simulink model "SRM"  (R2013b)
settings: Solver=ode8  StartTime=0.0  StopTime=2  FixedStep=Ts  RelTol=1e-3
InitFcn:
  | Iref=4
  | v_4dc = 78;
  | kp_speed =500;
  | ki_speed = 60;
  | sat_speed = 10;
  | x = 0.8 ;%%firing angle
  | kp_controller = 200;
  | ki_controller = 60;
  | ts = 1/10e4;
  | Ts = 1e-06;
undefined symbols (not defined in the file): find_system
libraries: simulink x1, powerlib x1
settings Model: Creator=Mircea Ruba  LastModifiedBy=agie
settings DataIOCC: SignalLoggingSaveFormat=ModelDataLogs
settings OptimizationCC: ExpressionDepthLimit=2147483647
settings DebuggingCC: FcnCallInpInsideContextMsg=UseLocalSettings  UnconnectedInputMsg=none  UnconnectedOutputMsg=none  UnconnectedLineMsg=none  StateNameClashWarn=warning
settings GRTTargetCC: CombineOutputUpdateFcns=off  GRTInterface=on
settings ConfigurationSet: Description=SimMechanics 2G

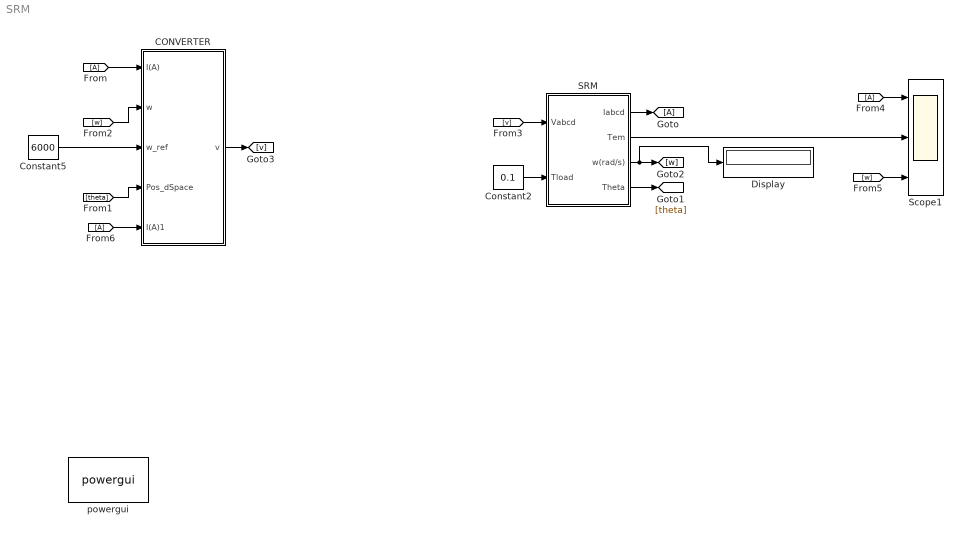
== system SRM ==
  CONVERTER : Subsystem  LoadFcn=find_system(gcs,'FollowLinks', 'on', 'LookUnderMasks', 'all');
  Constant2 : Constant  Value=0.1
  Constant5 : Constant  Value=6000
  Display : Display
  SRM : Subsystem
  Scope1 : Scope  NumInputPorts=3
      settings: TimeRange=0.5  YMin=-1~5.55112e-17~0  YMax=12~1~1100
  powergui : powerlib/powergui  Priority=2  SimulationMode=Discrete  SolverType=Tustin  SampleTime=Ts  frequency=60  SPID=off  DisableSnubberDevices=off  DisableRonSwitches=off  DisableVfSwitches=off  SwTol=0  Interpol=off  DisplayEquations=off  frequencyindice=0  Pbase=100e6  ErrMax=1e-4  Iterations=50  UnitsV=kV  UnitsW=MW  FunctionMessages=off  echomessages=off  HookPort=off  EnableUseOfTLC=off  x0status=blocks  RestoreLinks=warning  ResistiveCurrentMeasurement=off  Frange=[0:2:500]  Ylog=off  Xlog=on  ShowGrid=off  save=off  variable=ZData  ZoomFFT=on  StartTime=0.0  cycles=1  DisplayStyle=1  fundamental=60  FreqAxis=off  MaxFrequency=1000  frequencyindicesteady=1  RmsSteady=1  display=off  Ts=0  methode=off
  wires:
  SRM/2(Tem) -> Scope1/2
  Constant2/1 -> SRM/2(Tload)
  Constant5/1 -> CONVERTER/3(w_ref)
  SRM/1(Iabcd) -> [A]
  [A] -> CONVERTER/1(I(A))
  SRM/4(Theta) -> [theta]
  [theta] -> CONVERTER/4(Pos_dSpace)
  SRM/3(w(rad/s)) -> Display/1, [w]
  [w] -> CONVERTER/2(w)
  CONVERTER/1(v) -> [v]
  [v] -> SRM/1(Vabcd)
  [A] -> Scope1/1
  [w] -> Scope1/3
  [A] -> CONVERTER/5(I(A)1)

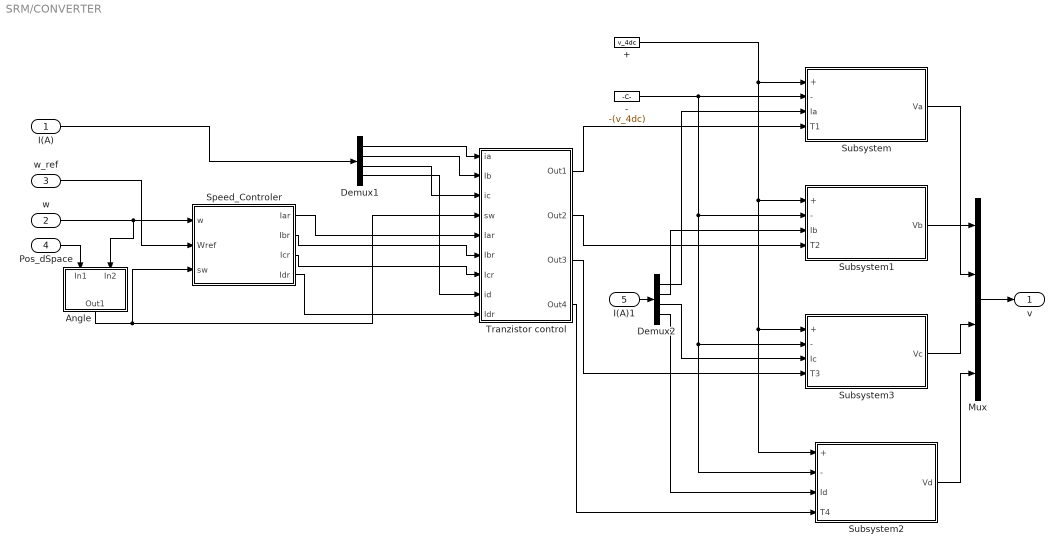
== system SRM/CONVERTER ==
  I(A) : Inport
  w : Inport  Port=2
  w_ref : Inport  Port=3
  Pos_dSpace : Inport  Port=4
  I(A)1 : Inport  Port=5
  + : Constant  Value=v_4dc
  - : Constant  Value=-(v_4dc)
  Angle : Subsystem
  Demux1 : Demux
  Demux2 : Demux
  Mux : Mux
  Speed_Controler : Subsystem
  Subsystem : Subsystem
  Subsystem1 : Subsystem
  Subsystem2 : Subsystem
  Subsystem3 : Subsystem
  Tranzistor control : Subsystem
  v : Outport
  wires:
  Demux1/4 -> Tranzistor control/8(id)
  Speed_Controler/4(Idr) -> Tranzistor control/9(Idr)
  Speed_Controler/1(Iar) -> Tranzistor control/5(Iar)
  Speed_Controler/2(Ibr) -> Tranzistor control/6(Ibr)
  Speed_Controler/3(Icr) -> Tranzistor control/7(Icr)
  Demux1/1 -> Tranzistor control/1(ia)
  Demux1/2 -> Tranzistor control/2(Ib)
  Demux1/3 -> Tranzistor control/3(ic)
  I(A)/1 -> Demux1/1
  w_ref/1 -> Speed_Controler/2(Wref)
  w/1 -> Speed_Controler/1(w), Angle/2(In2)
  Mux/1 -> v/1
  +/1 -> Subsystem2/1(+), Subsystem3/1(+), Subsystem1/1(+), Subsystem/1(+)
  -/1 -> Subsystem2/2(-), Subsystem3/2(-), Subsystem1/2(-), Subsystem/2(-)
  Angle/1(Out1) -> Speed_Controler/3("sw "), Tranzistor control/4("sw ")
  Pos_dSpace/1 -> Angle/1(In1)
  Tranzistor control/1(Out1) -> Subsystem/4(T1)
  Subsystem/1(Va) -> Mux/1
  Tranzistor control/2(Out2) -> Subsystem1/4(T2)
  Subsystem1/1(Vb) -> Mux/2
  Tranzistor control/4(Out4) -> Subsystem2/4(T4)
  Subsystem2/1(Vd) -> Mux/4
  Tranzistor control/3(Out3) -> Subsystem3/4(T3)
  Subsystem3/1(Vc) -> Mux/3
  I(A)1/1 -> Demux2/1
  Demux2/1 -> Subsystem/3(Ia)
  Demux2/2 -> Subsystem1/3(Ib)
  Demux2/3 -> Subsystem3/3(Ic)
  Demux2/4 -> Subsystem2/3(Id)

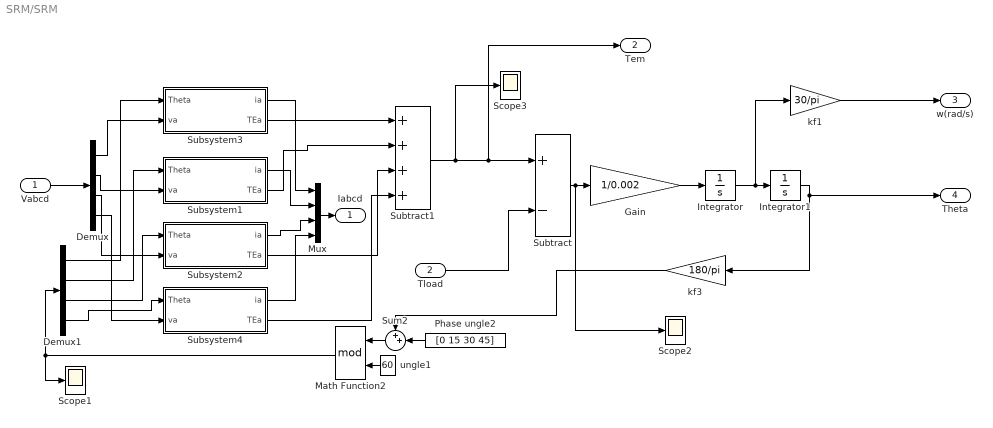
== system SRM/SRM ==
  Vabcd : Inport
  Tload : Inport  Port=2
  Demux : Demux
  Demux1 : Demux
  Gain : Gain  Gain=1/0.002
  Integrator : Integrator
  Integrator1 : Integrator  InitialCondition=10
  Math Function2 : Math  Operator=mod  SaturateOnIntegerOverflow=on
  Mux : Mux
  Phase ungle2 : Constant  Value=[0 15 30 45]
  Scope1 : Scope
      settings: TimeRange=0.4368  YMin=0  YMax=60
  Scope2 : Scope
      settings: TimeRange=0.4368  YMin=-550  YMax=300  SaveName=ScopeData11
  Scope3 : Scope
      settings: TimeRange=0.4368  YMin=-450  YMax=400  SaveName=ScopeData9
  Subsystem1 : Subsystem
  Subsystem2 : Subsystem
  Subsystem3 : Subsystem
  Subsystem4 : Subsystem
  Subtract : Sum  Inputs=+-
  Subtract1 : Sum  Inputs=++++
  Sum2 : Sum  Inputs=++|  SaturateOnIntegerOverflow=on  InputSameDT=on  OutDataTypeStr=Inherit: Same as first input
  kf1 : Gain  Gain=30/pi
  kf3 : Gain  Gain=180/pi
  ungle1 : Constant  Value=60
  Iabcd : Outport
  Tem : Outport  Port=2
  w(rad/s) : Outport  Port=3
  Theta : Outport  Port=4
  wires:
  Demux/4 -> Subsystem4/2(va)
  Demux1/4 -> Subsystem4/1(Theta)
  Subsystem4/2(TEa) -> Subtract1/4
  Subsystem4/1(ia) -> Mux/4
  Math Function2/1 -> Scope1/1, Demux1/1
  ungle1/1 -> Math Function2/2
  Sum2/1 -> Math Function2/1
  Phase ungle2/1 -> Sum2/2
  Vabcd/1 -> Demux/1
  Demux/1 -> Subsystem3/2(va)
  Mux/1 -> Iabcd/1
  Subsystem3/1(ia) -> Mux/1
  Subsystem1/1(ia) -> Mux/2
  Subsystem2/1(ia) -> Mux/3
  Subsystem2/2(TEa) -> Subtract1/3
  Subsystem1/2(TEa) -> Subtract1/2
  Subsystem3/2(TEa) -> Subtract1/1
  Subtract1/1 -> Subtract/1, Tem/1, Scope3/1
  Gain/1 -> Integrator/1
  Subtract/1 -> Scope2/1, Gain/1
  Integrator1/1 -> Theta/1, kf3/1
  Demux/2 -> Subsystem1/2(va)
  Demux/3 -> Subsystem2/2(va)
  Tload/1 -> Subtract/2
  kf3/1 -> Sum2/1
  Demux1/1 -> Subsystem3/1(Theta)
  Demux1/2 -> Subsystem1/1(Theta)
  Demux1/3 -> Subsystem2/1(Theta)
  Integrator/1 -> kf1/1, Integrator1/1
  kf1/1 -> w(rad/s)/1

== system SRM/CONVERTER/Angle ==
  In1 : Inport
  In2 : Inport  Port=2
  360 : Subsystem
  Position : Subsystem
  angle : Subsystem
  Out1 : Outport
  wires:
  Position/1(sw) -> Out1/1
  angle/1(Theta_On(Alpha)) -> Position/2(On angle)
  angle/2(Theta_Off(Beta)) -> Position/3(Off angle)
  In1/1 -> 360/1(In1)
  In2/1 -> angle/1(n)
  360/1(Out1) -> Position/1(dSpace POSITION)

== system SRM/CONVERTER/Speed_Controler ==
  w : Inport
  Wref : Inport  Port=2
  "sw " : Inport  Port=3
  Add : Sum  Inputs=+-
  Demux : Demux
  PI+AntiWindup : Subsystem
  Product{,1..3} (4 alike) : Product
  Iar : Outport
  Ibr : Outport  Port=2
  Icr : Outport  Port=3
  Idr : Outport  Port=4
  wires:
  Product3/1 -> Idr/1
  PI+AntiWindup/1(Out) -> Product2/1, Product3/1, Product1/1, Product/1
  Demux/4 -> Product3/2
  w/1 -> Add/2
  Wref/1 -> Add/1
  Product/1 -> Iar/1
  "sw "/1 -> Demux/1
  Product1/1 -> Ibr/1
  Product2/1 -> Icr/1
  Add/1 -> PI+AntiWindup/1(In)
  Demux/1 -> Product/2
  Demux/2 -> Product1/2
  Demux/3 -> Product2/2

== system SRM/CONVERTER/Subsystem ==
  + : Inport
  - : Inport  Port=2
  Ia : Inport  Port=3
  T1 : Inport  Port=4
  Constant5 : Constant  Value=0
  Switch : Switch  Criteria=u2 > Threshold  SaturateOnIntegerOverflow=on  InputSameDT=on
  Switch5 : Switch  Criteria=u2 > Threshold  SaturateOnIntegerOverflow=on  InputSameDT=on
  Va : Outport
  wires:
  +/1 -> Switch/1
  Ia/1 -> Switch5/2
  -/1 -> Switch5/1
  T1/1 -> Switch/2
  Constant5/1 -> Switch5/3
  Switch5/1 -> Switch/3
  Switch/1 -> Va/1

== system SRM/CONVERTER/Subsystem1 ==
  + : Inport
  - : Inport  Port=2
  Ib : Inport  Port=3
  T2 : Inport  Port=4
  Constant2 : Constant  Value=0
  Switch1 : Switch  Criteria=u2 > Threshold  SaturateOnIntegerOverflow=on  InputSameDT=on
  Switch2 : Switch  Criteria=u2 > Threshold  SaturateOnIntegerOverflow=on  InputSameDT=on
  Vb : Outport
  wires:
  Switch2/1 -> Switch1/3
  Constant2/1 -> Switch2/3
  T2/1 -> Switch1/2
  Switch1/1 -> Vb/1
  Ib/1 -> Switch2/2
  -/1 -> Switch2/1
  +/1 -> Switch1/1

== system SRM/CONVERTER/Subsystem2 ==
  + : Inport
  - : Inport  Port=2
  Id : Inport  Port=3
  T4 : Inport  Port=4
  Constant4 : Constant  Value=0
  Switch6 : Switch  Criteria=u2 > Threshold  SaturateOnIntegerOverflow=on  InputSameDT=on
  Switch7 : Switch  Criteria=u2 > Threshold  SaturateOnIntegerOverflow=on  InputSameDT=on
  Vd : Outport
  wires:
  T4/1 -> Switch6/2
  Switch6/1 -> Vd/1
  Constant4/1 -> Switch7/3
  Switch7/1 -> Switch6/3
  +/1 -> Switch6/1
  Id/1 -> Switch7/2
  -/1 -> Switch7/1

== system SRM/CONVERTER/Subsystem3 ==
  + : Inport
  - : Inport  Port=2
  Ic : Inport  Port=3
  T3 : Inport  Port=4
  Constant3 : Constant  Value=0
  Switch3 : Switch  Criteria=u2 > Threshold  SaturateOnIntegerOverflow=on  InputSameDT=on
  Switch4 : Switch  Criteria=u2 > Threshold  SaturateOnIntegerOverflow=on  InputSameDT=on
  Vc : Outport
  wires:
  Ic/1 -> Switch4/2
  +/1 -> Switch3/1
  -/1 -> Switch4/1
  T3/1 -> Switch3/2
  Switch3/1 -> Vc/1
  Constant3/1 -> Switch4/3
  Switch4/1 -> Switch3/3

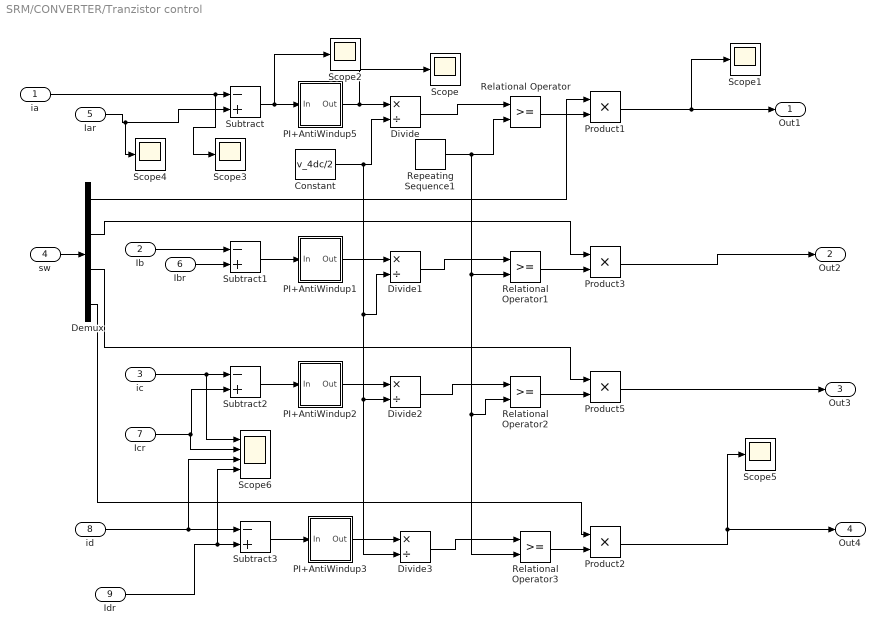
== system SRM/CONVERTER/Tranzistor control ==
  ia : Inport
  Ib : Inport  Port=2
  ic : Inport  Port=3
  "sw " : Inport  Port=4
  Iar : Inport  Port=5
  Ibr : Inport  Port=6
  Icr : Inport  Port=7
  id : Inport  Port=8
  Idr : Inport  Port=9
  Constant : Constant  Value=v_4dc/2
  Demux : Demux
  Divide{,1..3} (4 alike) : Product  Inputs=*/
  PI+AntiWindup1 : Subsystem
  PI+AntiWindup2 : Subsystem
  PI+AntiWindup3 : Subsystem
  PI+AntiWindup5 : Subsystem
  Product{1..3,5} (4 alike) : Product
  Relational Operator{,1..3} (4 alike) : RelationalOperator  OutDataTypeStr=boolean
  Repeating Sequence1 : simulink/Sources/Repeating Sequence  rep_seq_t=[0 0.5 1]*(1/10e3)  rep_seq_y=[-0.999 0.999 -0.999]
  Scope{,1..5} (6 alike) : Scope
      Scope settings: YMin=-45  YMax=45  SaveName=ScopeData10
      Scope1 settings: YMin=-45  YMax=45  SaveName=ScopeData16
      Scope2 settings: YMin=-5.5  YMax=5.5  SaveName=ScopeData17
      Scope3 settings: YMin=-0.008  YMax=-0.001  SaveName=ScopeData19
      Scope4 settings: YMin=-5.5  YMax=5.5  SaveName=ScopeData21
      Scope5 settings: YMin=-45  YMax=45  SaveName=ScopeData22
  Scope6 : Scope  NumInputPorts=4
      settings: YMin=-250~0~-80~0  YMax=50~5~10~5  SaveName=ScopeData23
  Subtract{,1..3} (4 alike) : Sum  Inputs=-+
  Out1 : Outport
  Out2 : Outport  Port=2
  Out3 : Outport  Port=3
  Out4 : Outport  Port=4
  wires:
  Product2/1 -> Scope5/1, Out4/1
  Constant/1 -> Divide/2, Divide3/2, Divide2/2, Divide1/2
  Divide3/1 -> Relational Operator3/1
  PI+AntiWindup3/1(Out) -> Divide3/1
  id/1 -> Scope6/3, Subtract3/1
  Idr/1 -> Scope6/4, Subtract3/2
  Subtract3/1 -> PI+AntiWindup3/1(In)
  Relational Operator3/1 -> Product2/2
  Demux/4 -> Product2/1
  Repeating Sequence1/1 -> Relational Operator/2, Relational Operator1/2, Relational Operator2/2, Relational Operator3/2
  Divide2/1 -> Relational Operator2/1
  PI+AntiWindup2/1(Out) -> Divide2/1
  Divide1/1 -> Relational Operator1/1
  PI+AntiWindup1/1(Out) -> Divide1/1
  PI+AntiWindup5/1(Out) -> Divide/1, Scope/1
  Divide/1 -> Relational Operator/1
  Iar/1 -> Scope4/1, Subtract/2
  Relational Operator/1 -> Product1/2
  Ib/1 -> Subtract1/1
  Ibr/1 -> Subtract1/2
  Subtract1/1 -> PI+AntiWindup1/1(In)
  Relational Operator1/1 -> Product3/2
  Product3/1 -> Out2/1
  ic/1 -> Scope6/1, Subtract2/1
  Icr/1 -> Scope6/2, Subtract2/2
  Subtract2/1 -> PI+AntiWindup2/1(In)
  Relational Operator2/1 -> Product5/2
  Product5/1 -> Out3/1
  Demux/1 -> Product1/1
  Demux/2 -> Product3/1
  Demux/3 -> Product5/1
  "sw "/1 -> Demux/1
  Product1/1 -> Scope1/1, Out1/1
  Subtract/1 -> Scope2/1, PI+AntiWindup5/1(In)
  ia/1 -> Scope3/1, Subtract/1

== system SRM/SRM/Subsystem1 ==
  Theta : Inport
  va : Inport  Port=2
  Gain : Gain  Gain=0.3
  Product : Product
  Product1 : Product
  Scope4 : Scope  NumInputPorts=3
      settings: TimeRange=0.5  YMin=-1~-1~-25  YMax=1~1~25  SaveName=ScopeData20
  "Subsystem2 " : Subsystem
  Sum : Sum  Inputs=|+-
  ia : Outport
  TEa : Outport  Port=2
  wires:
  va/1 -> Sum/1
  Sum/1 -> "Subsystem2 "/2(Lambda)
  "Subsystem2 "/2(Current) -> ia/1, Gain/1, Product1/2, Product1/1
  Gain/1 -> Sum/2
  Product1/1 -> Product/2, Scope4/2
  "Subsystem2 "/1(dL/dt) -> Product/1, Scope4/1
  Product/1 -> Scope4/3, TEa/1
  Theta/1 -> "Subsystem2 "/1(Theta)

== system SRM/SRM/Subsystem2 ==
  Theta : Inport
  va : Inport  Port=2
  Gain : Gain  Gain=0.3
  Product : Product
  Product1 : Product
  Scope4 : Scope  NumInputPorts=3
      settings: TimeRange=0.5  YMin=-1~-1~-25  YMax=1~1~25  SaveName=ScopeData20
  "Subsystem2 " : Subsystem
  Sum : Sum  Inputs=|+-
  ia : Outport
  TEa : Outport  Port=2
  wires:
  Theta/1 -> "Subsystem2 "/1(Theta)
  Product/1 -> TEa/1, Scope4/3
  "Subsystem2 "/1(dL/dt) -> Scope4/1, Product/1
  Product1/1 -> Product/2, Scope4/2
  Gain/1 -> Sum/2
  "Subsystem2 "/2(Current) -> Product1/1, Product1/2, Gain/1, ia/1
  Sum/1 -> "Subsystem2 "/2(Lambda)
  va/1 -> Sum/1

== system SRM/SRM/Subsystem3 ==
  Theta : Inport
  va : Inport  Port=2
  Gain : Gain  Gain=0.3
  Product : Product
  Product1 : Product
  "Subsystem2 " : Subsystem
  Sum : Sum  Inputs=|+-
  ia : Outport
  TEa : Outport  Port=2
  wires:
  Theta/1 -> "Subsystem2 "/1(Theta)
  Product/1 -> TEa/1
  "Subsystem2 "/1(dL/dt) -> Product/1
  Product1/1 -> Product/2
  Gain/1 -> Sum/2
  "Subsystem2 "/2(Current) -> Product1/1, Product1/2, Gain/1, ia/1
  Sum/1 -> "Subsystem2 "/2(Lambda)
  va/1 -> Sum/1

== system SRM/SRM/Subsystem4 ==
  Theta : Inport
  va : Inport  Port=2
  Gain : Gain
  Product : Product
  Product1 : Product
  Scope4 : Scope  NumInputPorts=3
      settings: TimeRange=0.5  YMin=-1~-1~-25  YMax=1~1~25  SaveName=ScopeData20
  "Subsystem2 " : Subsystem
  Sum : Sum  Inputs=|+-
  ia : Outport
  TEa : Outport  Port=2
  wires:
  va/1 -> Sum/1
  Sum/1 -> "Subsystem2 "/2(Lambda)
  "Subsystem2 "/2(Current) -> Scope4/2, ia/1, Gain/1, Product1/2, Product1/1
  Gain/1 -> Sum/2
  Product1/1 -> Product/2
  "Subsystem2 "/1(dL/dt) -> Scope4/1, Product/1
  Product/1 -> Scope4/3, TEa/1
  Theta/1 -> "Subsystem2 "/1(Theta)

== system SRM/CONVERTER/Angle/360 ==
  In1 : Inport
  Constant2 : Constant  Value=360
  Math Function2 : Math  Operator=mod  SaturateOnIntegerOverflow=on
  kf2 : Gain  Gain=180/pi
  Out1 : Outport
  wires:
  Constant2/1 -> Math Function2/2
  kf2/1 -> Math Function2/1
  Math Function2/1 -> Out1/1
  In1/1 -> kf2/1

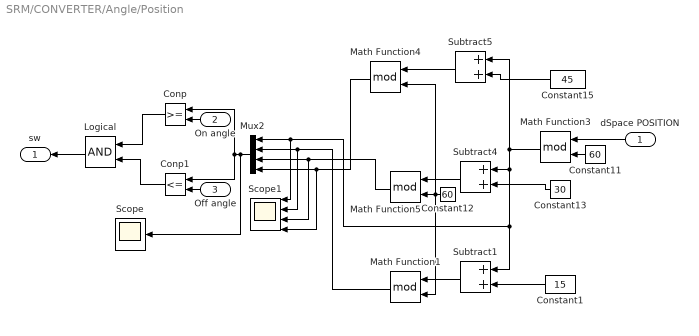
== system SRM/CONVERTER/Angle/Position ==
  dSpace POSITION : Inport
  On angle : Inport  Port=2
  Off angle : Inport  Port=3
  " Logical" : Logic  AllPortsSameDT=off  OutDataTypeStr=boolean
  Conp : RelationalOperator  OutDataTypeStr=boolean
  Conp1 : RelationalOperator  Operator=<=  OutDataTypeStr=boolean
  Constant1 : Constant  Value=15
  Constant11 : Constant  Value=60
  Constant12 : Constant  Value=60
  Constant13 : Constant  Value=30
  Constant15 : Constant  Value=45
  Math Function{1,3..5} (4 alike) : Math  Operator=mod  SaturateOnIntegerOverflow=on
  Mux2 : Mux
  Scope : Scope
      settings: YMin=10  YMax=75  SaveName=ScopeData14
  Scope1 : Scope  NumInputPorts=4
      settings: YMin=10~-5~-5~-5  YMax=75~5~5~5  SaveName=ScopeData3
  Subtract1 : Sum
  Subtract4 : Sum
  Subtract5 : Sum
  sw : Outport
  wires:
  Math Function1/1 -> Scope1/2, Mux2/2
  Constant1/1 -> Subtract1/2
  Subtract1/1 -> Math Function1/1
  Constant11/1 -> Math Function3/2
  Math Function3/1 -> Subtract1/1, Mux2/1, Scope1/1, Subtract4/1, Subtract5/1
  Subtract4/1 -> Math Function5/1
  Constant13/1 -> Subtract4/2
  Subtract5/1 -> Math Function4/1
  dSpace POSITION/1 -> Math Function3/1
  Constant15/1 -> Subtract5/2
  Math Function4/1 -> Mux2/4, Scope1/4
  Constant12/1 -> Math Function4/2, Math Function5/2, Math Function1/2
  Math Function5/1 -> Mux2/3, Scope1/3
  Mux2/1 -> Scope/1, Conp/1, Conp1/1
  Conp/1 -> " Logical"/1
  Conp1/1 -> " Logical"/2
  " Logical"/1 -> sw/1
  On angle/1 -> Conp/2
  Off angle/1 -> Conp1/2

== system SRM/CONVERTER/Angle/angle ==
  n : Inport
  Iref1 : Constant  Value=Iref
  Subsystem : Subsystem
  Subsystem1 : Subsystem
  Theta_On(Alpha) : Outport
  Theta_Off(Beta) : Outport  Port=2
  wires:
  Subsystem/1(Theta_ON) -> Theta_On(Alpha)/1
  Subsystem1/1(Theta_Off) -> Theta_Off(Beta)/1
  Iref1/1 -> Subsystem1/1(Iref), Subsystem/1(Iref)
  n/1 -> Subsystem1/2(n), Subsystem/2(n)

== system SRM/CONVERTER/Speed_Controler/PI+AntiWindup ==
  In : Inport
  Gain10 : Gain  Gain=ki_speed
  Gain11 : Gain  Gain=1/kp_speed
  Gain9 : Gain  Gain=kp_speed
  Integrator3 : Integrator
  Saturation3 : Saturate  UpperLimit=sat_speed  LowerLimit=-sat_speed
  Sum10 : Sum  Inputs=|++
  Sum11 : Sum  Inputs=-+|
  Sum9 : Sum
  Out : Outport
  wires:
  Sum9/1 -> Integrator3/1
  Integrator3/1 -> Gain10/1
  Gain9/1 -> Sum10/1
  Sum11/1 -> Gain11/1
  In/1 -> Sum9/1, Gain9/1
  Saturation3/1 -> Out/1, Sum11/2
  Sum10/1 -> Saturation3/1, Sum11/1
  Gain11/1 -> Sum9/2
  Gain10/1 -> Sum10/2

== system SRM/CONVERTER/Tranzistor control/PI+AntiWindup1 ==
  In : Inport
  Gain10 : Gain  Gain=ki_controller
  Gain11 : Gain  Gain=1/kp_controller
  Gain9 : Gain  Gain=kp_controller
  Integrator3 : Integrator
  Saturation3 : Saturate  UpperLimit=v_4dc/2  LowerLimit=-v_4dc/2  LinearizeAsGain=off
  Sum10 : Sum  Inputs=|++
  Sum11 : Sum  Inputs=-+|
  Sum9 : Sum
  Out : Outport
  wires:
  Gain11/1 -> Sum9/2
  In/1 -> Gain9/1, Sum9/1
  Sum11/1 -> Gain11/1
  Sum10/1 -> Saturation3/1, Sum11/1
  Gain9/1 -> Sum10/1
  Gain10/1 -> Sum10/2
  Integrator3/1 -> Gain10/1
  Sum9/1 -> Integrator3/1
  Saturation3/1 -> Sum11/2, Out/1

== system SRM/CONVERTER/Tranzistor control/PI+AntiWindup2 ==
  In : Inport
  Gain10 : Gain  Gain=ki_controller
  Gain11 : Gain  Gain=1/kp_controller
  Gain9 : Gain  Gain=kp_controller
  Integrator3 : Integrator
  Saturation3 : Saturate  UpperLimit=v_4dc/2  LowerLimit=-v_4dc/2  LinearizeAsGain=off
  Sum10 : Sum  Inputs=|++
  Sum11 : Sum  Inputs=-+|
  Sum9 : Sum
  Out : Outport
  wires:
  Saturation3/1 -> Out/1, Sum11/2
  Sum9/1 -> Integrator3/1
  Integrator3/1 -> Gain10/1
  Gain10/1 -> Sum10/2
  Gain9/1 -> Sum10/1
  Sum10/1 -> Saturation3/1, Sum11/1
  Sum11/1 -> Gain11/1
  In/1 -> Sum9/1, Gain9/1
  Gain11/1 -> Sum9/2

== system SRM/CONVERTER/Tranzistor control/PI+AntiWindup3 ==
  In : Inport
  Gain10 : Gain  Gain=ki_controller
  Gain11 : Gain  Gain=1/kp_controller
  Gain9 : Gain  Gain=kp_controller
  Integrator3 : Integrator
  Saturation3 : Saturate  UpperLimit=v_4dc/2  LowerLimit=-v_4dc/2  LinearizeAsGain=off
  Sum10 : Sum  Inputs=|++
  Sum11 : Sum  Inputs=-+|
  Sum9 : Sum
  Out : Outport
  wires:
  Saturation3/1 -> Out/1, Sum11/2
  Sum9/1 -> Integrator3/1
  Integrator3/1 -> Gain10/1
  Gain10/1 -> Sum10/2
  Gain9/1 -> Sum10/1
  Sum10/1 -> Saturation3/1, Sum11/1
  Sum11/1 -> Gain11/1
  In/1 -> Sum9/1, Gain9/1
  Gain11/1 -> Sum9/2

== system SRM/CONVERTER/Tranzistor control/PI+AntiWindup5 ==
  In : Inport
  Gain10 : Gain  Gain=ki_controller
  Gain11 : Gain  Gain=1/kp_controller
  Gain9 : Gain  Gain=kp_controller
  Integrator3 : Integrator
  Saturation3 : Saturate  UpperLimit=v_4dc/2  LowerLimit=-v_4dc/2  LinearizeAsGain=off
  Scope : Scope  NumInputPorts=4
      settings: YMin=-5~-5000~0.2~-1500  YMax=5~45000~0.65~250  SaveName=ScopeData4
  Sum10 : Sum  Inputs=|++
  Sum11 : Sum  Inputs=-+|
  Sum9 : Sum
  Out : Outport
  wires:
  Saturation3/1 -> Scope/1, Out/1, Sum11/2
  Sum9/1 -> Integrator3/1
  Integrator3/1 -> Gain10/1
  Gain10/1 -> Sum10/2, Scope/4
  Gain9/1 -> Scope/3, Sum10/1
  Sum10/1 -> Scope/2, Saturation3/1, Sum11/1
  Sum11/1 -> Gain11/1
  In/1 -> Sum9/1, Gain9/1
  Gain11/1 -> Sum9/2

== system SRM/SRM/Subsystem1/Subsystem2  ==
  Theta : Inport
  Lambda : Inport  Port=2
  Divide : Product  Inputs=*/
  Integrator : Integrator
  Subsystem1 : Subsystem
  Subsystem2 : Subsystem
  dL/dt : Outport
  Current : Outport  Port=2
  wires:
  Subsystem1/1(dL/dt) -> dL/dt/1
  Theta/1 -> Subsystem2/1(Theta), Subsystem1/1(Theta)
  Lambda/1 -> Divide/1
  Subsystem2/1(L(theta)) -> Divide/2
  Divide/1 -> Integrator/1
  Integrator/1 -> Current/1

== system SRM/SRM/Subsystem2/Subsystem2  ==
  Theta : Inport
  Lambda : Inport  Port=2
  Divide : Product  Inputs=*/
  Integrator : Integrator
  Subsystem1 : Subsystem
  Subsystem2 : Subsystem
  dL/dt : Outport
  Current : Outport  Port=2
  wires:
  Divide/1 -> Integrator/1
  Subsystem2/1(L(theta)) -> Divide/2
  Lambda/1 -> Divide/1
  Theta/1 -> Subsystem1/1(Theta), Subsystem2/1(Theta)
  Subsystem1/1(dL/dt) -> dL/dt/1
  Integrator/1 -> Current/1

== system SRM/SRM/Subsystem3/Subsystem2  ==
  Theta : Inport
  Lambda : Inport  Port=2
  Divide : Product  Inputs=*/
  Integrator1 : Integrator
  Subsystem1 : Subsystem
  Subsystem2 : Subsystem
  dL/dt : Outport
  Current : Outport  Port=2
  wires:
  Divide/1 -> Integrator1/1
  Subsystem2/1(L(theta)) -> Divide/2
  Lambda/1 -> Divide/1
  Theta/1 -> Subsystem1/1(Theta), Subsystem2/1(Theta)
  Subsystem1/1(dL/dt) -> dL/dt/1
  Integrator1/1 -> Current/1

== system SRM/SRM/Subsystem4/Subsystem2  ==
  Theta : Inport
  Lambda : Inport  Port=2
  Divide : Product  Inputs=*/
  Integrator : Integrator
  Subsystem1 : Subsystem
  Subsystem2 : Subsystem
  dL/dt : Outport
  Current : Outport  Port=2
  wires:
  Subsystem1/1(dL/dt) -> dL/dt/1
  Theta/1 -> Subsystem2/1(Theta), Subsystem1/1(Theta)
  Lambda/1 -> Divide/1
  Subsystem2/1(L(theta)) -> Divide/2
  Divide/1 -> Integrator/1
  Integrator/1 -> Current/1

== system SRM/CONVERTER/Angle/angle/Subsystem ==
  Iref : Inport
  n : Inport  Port=2
  Dc link : Constant  Value=42
  Divide : Product  Inputs=*/
  Lu : Constant  Value=0.00053
  Product : Product
  Product1 : Product
  Product2 : Product
  Subtract : Sum  Inputs=+-
  Theta_m : Constant  Value=15
  ct : Constant  Value=8
  Theta_ON : Outport
  wires:
  Theta_m/1 -> Subtract/1
  ct/1 -> Product/1
  Product1/1 -> Product/2
  Product/1 -> Product2/1
  Product2/1 -> Divide/1
  Dc link/1 -> Divide/2
  Divide/1 -> Subtract/2
  Subtract/1 -> Theta_ON/1
  n/1 -> Product1/1
  Lu/1 -> Product1/2
  Iref/1 -> Product2/2

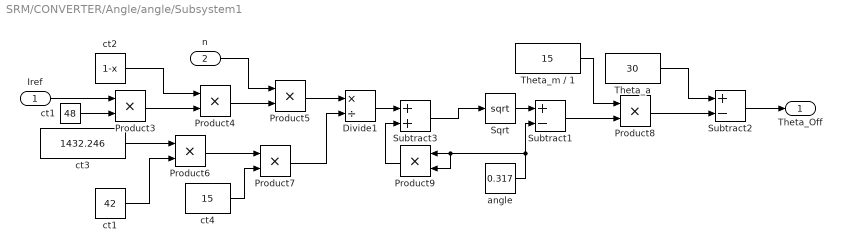
== system SRM/CONVERTER/Angle/angle/Subsystem1 ==
  Iref : Inport
  n : Inport  Port=2
  Divide1 : Product  Inputs=*/
  Product{3..9} (7 alike) : Product
  Sqrt : Sqrt  SaturateOnIntegerOverflow=on
  Subtract1 : Sum  Inputs=+-
  Subtract2 : Sum  Inputs=+-
  Subtract3 : Sum
  Theta_a : Constant  Value=30
  Theta_m / 1 : Constant  Value=15
  angle : Constant  Value=0.317
  ct1 : Constant  Value=42
  "ct1 " : Constant  Value=48
  ct2 : Constant  Value=1-x
  ct3 : Constant  Value=1432.246
  ct4 : Constant  Value=15
  Theta_Off : Outport
  wires:
  "ct1 "/1 -> Product3/2
  Product3/1 -> Product4/2
  ct2/1 -> Product4/1
  Product4/1 -> Product5/2
  n/1 -> Product5/1
  ct3/1 -> Product6/1
  ct1/1 -> Product6/2
  Product6/1 -> Product7/1
  ct4/1 -> Product7/2
  Product5/1 -> Divide1/1
  Product7/1 -> Divide1/2
  Sqrt/1 -> Subtract1/1
  angle/1 -> Product9/2, Product9/1, Subtract1/2
  Subtract1/1 -> Product8/2
  Theta_m / 1/1 -> Product8/1
  Product8/1 -> Subtract2/2
  Theta_a/1 -> Subtract2/1
  Subtract2/1 -> Theta_Off/1
  Divide1/1 -> Subtract3/1
  Subtract3/1 -> Sqrt/1
  Product9/1 -> Subtract3/2
  Iref/1 -> Product3/1

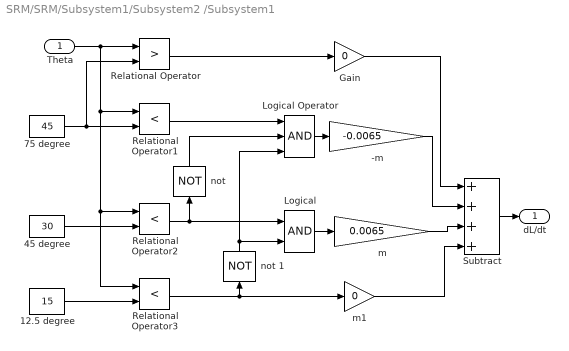
== system SRM/SRM/Subsystem1/Subsystem2 /Subsystem1 ==
  Theta : Inport
  -m : Gain  Gain=-0.0065
  12.5 degree : Constant  Value=15
  45 degree : Constant  Value=30
  75 degree : Constant  Value=45
  Gain : Gain  Gain=0
  Logical : Logic  AllPortsSameDT=off  OutDataTypeStr=boolean
  Logical Operator : Logic  Inputs=3  AllPortsSameDT=off  OutDataTypeStr=boolean
  Relational Operator : RelationalOperator  Operator=>  OutDataTypeStr=boolean
  Relational Operator1 : RelationalOperator  Operator=<  OutDataTypeStr=boolean
  Relational Operator2 : RelationalOperator  Operator=<  OutDataTypeStr=boolean
  Relational Operator3 : RelationalOperator  Operator=<  OutDataTypeStr=boolean
  Subtract : Sum  Inputs=++++
  m : Gain  Gain=0.0065
  m1 : Gain  Gain=0
  "not " : Logic  Operator=NOT  AllPortsSameDT=off  OutDataTypeStr=boolean
  not 1 : Logic  Operator=NOT  AllPortsSameDT=off  OutDataTypeStr=boolean
  dL/dt : Outport
  wires:
  75 degree/1 -> Relational Operator/2, Relational Operator1/2
  45 degree/1 -> Relational Operator2/2
  12.5 degree/1 -> Relational Operator3/2
  Relational Operator1/1 -> Logical Operator/1
  Relational Operator3/1 -> m1/1, not 1/1
  "not "/1 -> Logical Operator/2
  not 1/1 -> Logical/2, Logical Operator/3
  Relational Operator2/1 -> Logical/1, "not "/1
  Theta/1 -> Relational Operator2/1, Relational Operator3/1, Relational Operator1/1, Relational Operator/1
  Subtract/1 -> dL/dt/1
  Relational Operator/1 -> Gain/1
  Gain/1 -> Subtract/1
  Logical Operator/1 -> -m/1
  -m/1 -> Subtract/2
  Logical/1 -> m/1
  m/1 -> Subtract/3
  m1/1 -> Subtract/4

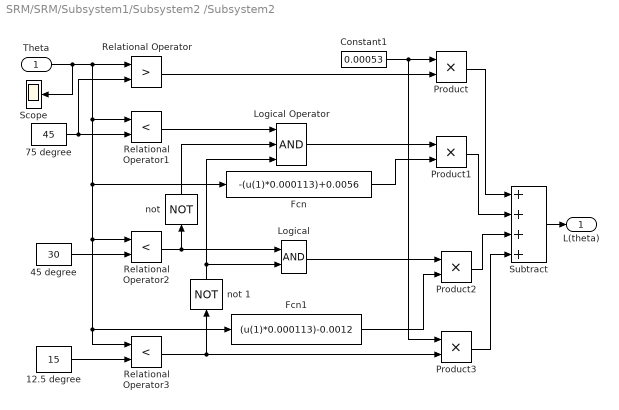
== system SRM/SRM/Subsystem1/Subsystem2 /Subsystem2 ==
  Theta : Inport
  12.5 degree : Constant  Value=15
  45 degree : Constant  Value=30
  75 degree : Constant  Value=45
  Constant1 : Constant  Value=0.00053
  Fcn : Fcn  Expr=-(u(1)*0.000113)+0.0056
  Fcn1 : Fcn  Expr=(u(1)*0.000113)-0.0012
  Logical : Logic  AllPortsSameDT=off  OutDataTypeStr=boolean
  Logical Operator : Logic  Inputs=3  AllPortsSameDT=off  OutDataTypeStr=boolean
  Product{,1..3} (4 alike) : Product
  Relational Operator : RelationalOperator  Operator=>  OutDataTypeStr=boolean
  Relational Operator1 : RelationalOperator  Operator=<  OutDataTypeStr=boolean
  Relational Operator2 : RelationalOperator  Operator=<  OutDataTypeStr=boolean
  Relational Operator3 : RelationalOperator  Operator=<  OutDataTypeStr=boolean
  Scope : Scope
      settings: YMin=-10  YMax=10  SaveName=ScopeData8
  Subtract : Sum  Inputs=++++
  "not " : Logic  Operator=NOT  AllPortsSameDT=off  OutDataTypeStr=boolean
  not 1 : Logic  Operator=NOT  AllPortsSameDT=off  OutDataTypeStr=boolean
  L(theta) : Outport
  wires:
  Subtract/1 -> L(theta)/1
  Product3/1 -> Subtract/4
  Product2/1 -> Subtract/3
  Product1/1 -> Subtract/2
  Product/1 -> Subtract/1
  Fcn1/1 -> Product2/2
  Theta/1 -> Relational Operator/1, Relational Operator1/1, Fcn/1, Relational Operator3/1, Fcn1/1, Relational Operator2/1, Scope/1
  Logical/1 -> Product2/1
  Fcn/1 -> Product1/2
  Logical Operator/1 -> Product1/1
  Relational Operator2/1 -> "not "/1, Logical/1
  not 1/1 -> Logical/2, Logical Operator/3
  "not "/1 -> Logical Operator/2
  Relational Operator3/1 -> not 1/1, Product3/2
  Relational Operator1/1 -> Logical Operator/1
  12.5 degree/1 -> Relational Operator3/2
  45 degree/1 -> Relational Operator2/2
  Constant1/1 -> Product/1, Product3/1
  Relational Operator/1 -> Product/2
  75 degree/1 -> Relational Operator1/2, Relational Operator/2

== system SRM/SRM/Subsystem2/Subsystem2 /Subsystem1 ==
  Theta : Inport
  -m : Gain  Gain=-0.0065
  12.5 degree : Constant  Value=15
  45 degree : Constant  Value=30
  75 degree : Constant  Value=45
  Gain : Gain  Gain=0
  Logical : Logic  AllPortsSameDT=off  OutDataTypeStr=boolean
  Logical Operator : Logic  Inputs=3  AllPortsSameDT=off  OutDataTypeStr=boolean
  Relational Operator : RelationalOperator  Operator=>  OutDataTypeStr=boolean
  Relational Operator1 : RelationalOperator  Operator=<  OutDataTypeStr=boolean
  Relational Operator2 : RelationalOperator  Operator=<  OutDataTypeStr=boolean
  Relational Operator3 : RelationalOperator  Operator=<  OutDataTypeStr=boolean
  Subtract : Sum  Inputs=++++
  m : Gain  Gain=0.0065
  m1 : Gain  Gain=0
  "not " : Logic  Operator=NOT  AllPortsSameDT=off  OutDataTypeStr=boolean
  not 1 : Logic  Operator=NOT  AllPortsSameDT=off  OutDataTypeStr=boolean
  dL/dt : Outport
  wires:
  m1/1 -> Subtract/4
  m/1 -> Subtract/3
  Logical/1 -> m/1
  -m/1 -> Subtract/2
  Logical Operator/1 -> -m/1
  Gain/1 -> Subtract/1
  Relational Operator/1 -> Gain/1
  Subtract/1 -> dL/dt/1
  Theta/1 -> Relational Operator/1, Relational Operator1/1, Relational Operator3/1, Relational Operator2/1
  Relational Operator2/1 -> "not "/1, Logical/1
  not 1/1 -> Logical Operator/3, Logical/2
  "not "/1 -> Logical Operator/2
  Relational Operator3/1 -> not 1/1, m1/1
  Relational Operator1/1 -> Logical Operator/1
  12.5 degree/1 -> Relational Operator3/2
  45 degree/1 -> Relational Operator2/2
  75 degree/1 -> Relational Operator1/2, Relational Operator/2

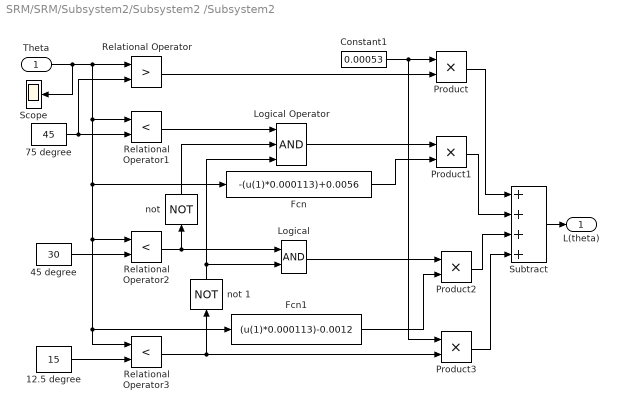
== system SRM/SRM/Subsystem2/Subsystem2 /Subsystem2 ==
  Theta : Inport
  12.5 degree : Constant  Value=15
  45 degree : Constant  Value=30
  75 degree : Constant  Value=45
  Constant1 : Constant  Value=0.00053
  Fcn : Fcn  Expr=-(u(1)*0.000113)+0.0056
  Fcn1 : Fcn  Expr=(u(1)*0.000113)-0.0012
  Logical : Logic  AllPortsSameDT=off  OutDataTypeStr=boolean
  Logical Operator : Logic  Inputs=3  AllPortsSameDT=off  OutDataTypeStr=boolean
  Product{,1..3} (4 alike) : Product
  Relational Operator : RelationalOperator  Operator=>  OutDataTypeStr=boolean
  Relational Operator1 : RelationalOperator  Operator=<  OutDataTypeStr=boolean
  Relational Operator2 : RelationalOperator  Operator=<  OutDataTypeStr=boolean
  Relational Operator3 : RelationalOperator  Operator=<  OutDataTypeStr=boolean
  Scope : Scope
      settings: YMin=-10  YMax=10  SaveName=ScopeData8
  Subtract : Sum  Inputs=++++
  "not " : Logic  Operator=NOT  AllPortsSameDT=off  OutDataTypeStr=boolean
  not 1 : Logic  Operator=NOT  AllPortsSameDT=off  OutDataTypeStr=boolean
  L(theta) : Outport
  wires:
  75 degree/1 -> Relational Operator/2, Relational Operator1/2
  Relational Operator/1 -> Product/2
  Constant1/1 -> Product3/1, Product/1
  45 degree/1 -> Relational Operator2/2
  12.5 degree/1 -> Relational Operator3/2
  Relational Operator1/1 -> Logical Operator/1
  Relational Operator3/1 -> Product3/2, not 1/1
  "not "/1 -> Logical Operator/2
  not 1/1 -> Logical Operator/3, Logical/2
  Relational Operator2/1 -> Logical/1, "not "/1
  Logical Operator/1 -> Product1/1
  Fcn/1 -> Product1/2
  Logical/1 -> Product2/1
  Theta/1 -> Scope/1, Relational Operator2/1, Fcn1/1, Relational Operator3/1, Fcn/1, Relational Operator1/1, Relational Operator/1
  Fcn1/1 -> Product2/2
  Product/1 -> Subtract/1
  Product1/1 -> Subtract/2
  Product2/1 -> Subtract/3
  Product3/1 -> Subtract/4
  Subtract/1 -> L(theta)/1

== system SRM/SRM/Subsystem3/Subsystem2 /Subsystem1 ==
  Theta : Inport
  -m : Gain  Gain=-0.0065
  12.5 degree : Constant  Value=15
  45 degree : Constant  Value=30
  75 degree : Constant  Value=45
  Gain : Gain  Gain=0
  Logical : Logic  AllPortsSameDT=off  OutDataTypeStr=boolean
  Logical Operator : Logic  Inputs=3  AllPortsSameDT=off  OutDataTypeStr=boolean
  Relational Operator : RelationalOperator  Operator=>  OutDataTypeStr=boolean
  Relational Operator1 : RelationalOperator  Operator=<  OutDataTypeStr=boolean
  Relational Operator2 : RelationalOperator  Operator=<  OutDataTypeStr=boolean
  Relational Operator3 : RelationalOperator  Operator=<  OutDataTypeStr=boolean
  Subtract : Sum  Inputs=++++
  m : Gain  Gain=0.0065
  m1 : Gain  Gain=0
  "not " : Logic  Operator=NOT  AllPortsSameDT=off  OutDataTypeStr=boolean
  not 1 : Logic  Operator=NOT  AllPortsSameDT=off  OutDataTypeStr=boolean
  dL/dt : Outport
  wires:
  m1/1 -> Subtract/4
  m/1 -> Subtract/3
  Logical/1 -> m/1
  -m/1 -> Subtract/2
  Logical Operator/1 -> -m/1
  Gain/1 -> Subtract/1
  Relational Operator/1 -> Gain/1
  Subtract/1 -> dL/dt/1
  Theta/1 -> Relational Operator/1, Relational Operator1/1, Relational Operator3/1, Relational Operator2/1
  Relational Operator2/1 -> "not "/1, Logical/1
  not 1/1 -> Logical Operator/3, Logical/2
  "not "/1 -> Logical Operator/2
  Relational Operator3/1 -> not 1/1, m1/1
  Relational Operator1/1 -> Logical Operator/1
  12.5 degree/1 -> Relational Operator3/2
  45 degree/1 -> Relational Operator2/2
  75 degree/1 -> Relational Operator1/2, Relational Operator/2

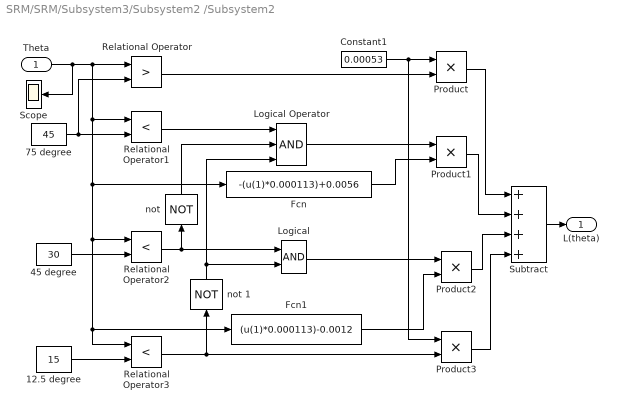
== system SRM/SRM/Subsystem3/Subsystem2 /Subsystem2 ==
  Theta : Inport
  12.5 degree : Constant  Value=15
  45 degree : Constant  Value=30
  75 degree : Constant  Value=45
  Constant1 : Constant  Value=0.00053
  Fcn : Fcn  Expr=-(u(1)*0.000113)+0.0056
  Fcn1 : Fcn  Expr=(u(1)*0.000113)-0.0012
  Logical : Logic  AllPortsSameDT=off  OutDataTypeStr=boolean
  Logical Operator : Logic  Inputs=3  AllPortsSameDT=off  OutDataTypeStr=boolean
  Product{,1..3} (4 alike) : Product
  Relational Operator : RelationalOperator  Operator=>  OutDataTypeStr=boolean
  Relational Operator1 : RelationalOperator  Operator=<  OutDataTypeStr=boolean
  Relational Operator2 : RelationalOperator  Operator=<  OutDataTypeStr=boolean
  Relational Operator3 : RelationalOperator  Operator=<  OutDataTypeStr=boolean
  Scope : Scope
      settings: YMin=-10  YMax=10  SaveName=ScopeData8
  Subtract : Sum  Inputs=++++
  "not " : Logic  Operator=NOT  AllPortsSameDT=off  OutDataTypeStr=boolean
  not 1 : Logic  Operator=NOT  AllPortsSameDT=off  OutDataTypeStr=boolean
  L(theta) : Outport
  wires:
  75 degree/1 -> Relational Operator/2, Relational Operator1/2
  Relational Operator/1 -> Product/2
  Constant1/1 -> Product3/1, Product/1
  45 degree/1 -> Relational Operator2/2
  12.5 degree/1 -> Relational Operator3/2
  Relational Operator1/1 -> Logical Operator/1
  Relational Operator3/1 -> Product3/2, not 1/1
  "not "/1 -> Logical Operator/2
  not 1/1 -> Logical Operator/3, Logical/2
  Relational Operator2/1 -> Logical/1, "not "/1
  Logical Operator/1 -> Product1/1
  Fcn/1 -> Product1/2
  Logical/1 -> Product2/1
  Theta/1 -> Scope/1, Relational Operator2/1, Fcn1/1, Relational Operator3/1, Fcn/1, Relational Operator1/1, Relational Operator/1
  Fcn1/1 -> Product2/2
  Product/1 -> Subtract/1
  Product1/1 -> Subtract/2
  Product2/1 -> Subtract/3
  Product3/1 -> Subtract/4
  Subtract/1 -> L(theta)/1

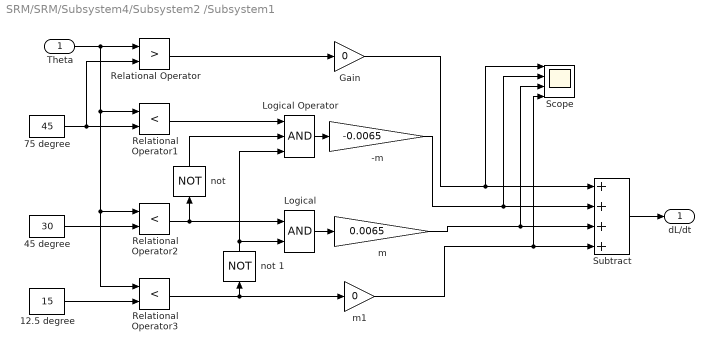
== system SRM/SRM/Subsystem4/Subsystem2 /Subsystem1 ==
  Theta : Inport
  -m : Gain  Gain=-0.0065
  12.5 degree : Constant  Value=15
  45 degree : Constant  Value=30
  75 degree : Constant  Value=45
  Gain : Gain  Gain=0
  Logical : Logic  AllPortsSameDT=off  OutDataTypeStr=boolean
  Logical Operator : Logic  Inputs=3  AllPortsSameDT=off  OutDataTypeStr=boolean
  Relational Operator : RelationalOperator  Operator=>  OutDataTypeStr=boolean
  Relational Operator1 : RelationalOperator  Operator=<  OutDataTypeStr=boolean
  Relational Operator2 : RelationalOperator  Operator=<  OutDataTypeStr=boolean
  Relational Operator3 : RelationalOperator  Operator=<  OutDataTypeStr=boolean
  Scope : Scope  NumInputPorts=4
      settings: YMin=0~-0.007~0~0  YMax=1~0~0.007~1  SaveName=ScopeData5
  Subtract : Sum  Inputs=++++
  m : Gain  Gain=0.0065
  m1 : Gain  Gain=0
  "not " : Logic  Operator=NOT  AllPortsSameDT=off  OutDataTypeStr=boolean
  not 1 : Logic  Operator=NOT  AllPortsSameDT=off  OutDataTypeStr=boolean
  dL/dt : Outport
  wires:
  75 degree/1 -> Relational Operator/2, Relational Operator1/2
  45 degree/1 -> Relational Operator2/2
  12.5 degree/1 -> Relational Operator3/2
  Relational Operator1/1 -> Logical Operator/1
  Relational Operator3/1 -> m1/1, not 1/1
  "not "/1 -> Logical Operator/2
  not 1/1 -> Logical/2, Logical Operator/3
  Relational Operator2/1 -> Logical/1, "not "/1
  Theta/1 -> Relational Operator2/1, Relational Operator3/1, Relational Operator1/1, Relational Operator/1
  Subtract/1 -> dL/dt/1
  Relational Operator/1 -> Gain/1
  Gain/1 -> Scope/1, Subtract/1
  Logical Operator/1 -> -m/1
  -m/1 -> Scope/2, Subtract/2
  Logical/1 -> m/1
  m/1 -> Scope/3, Subtract/3
  m1/1 -> Scope/4, Subtract/4

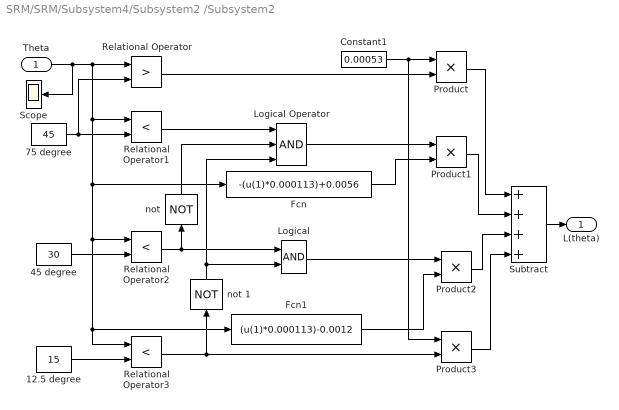
== system SRM/SRM/Subsystem4/Subsystem2 /Subsystem2 ==
  Theta : Inport
  12.5 degree : Constant  Value=15
  45 degree : Constant  Value=30
  75 degree : Constant  Value=45
  Constant1 : Constant  Value=0.00053
  Fcn : Fcn  Expr=-(u(1)*0.000113)+0.0056
  Fcn1 : Fcn  Expr=(u(1)*0.000113)-0.0012
  Logical : Logic  AllPortsSameDT=off  OutDataTypeStr=boolean
  Logical Operator : Logic  Inputs=3  AllPortsSameDT=off  OutDataTypeStr=boolean
  Product{,1..3} (4 alike) : Product
  Relational Operator : RelationalOperator  Operator=>  OutDataTypeStr=boolean
  Relational Operator1 : RelationalOperator  Operator=<  OutDataTypeStr=boolean
  Relational Operator2 : RelationalOperator  Operator=<  OutDataTypeStr=boolean
  Relational Operator3 : RelationalOperator  Operator=<  OutDataTypeStr=boolean
  Scope : Scope
      settings: YMin=-10  YMax=10  SaveName=ScopeData8
  Subtract : Sum  Inputs=++++
  "not " : Logic  Operator=NOT  AllPortsSameDT=off  OutDataTypeStr=boolean
  not 1 : Logic  Operator=NOT  AllPortsSameDT=off  OutDataTypeStr=boolean
  L(theta) : Outport
  wires:
  Subtract/1 -> L(theta)/1
  Product3/1 -> Subtract/4
  Product2/1 -> Subtract/3
  Product1/1 -> Subtract/2
  Product/1 -> Subtract/1
  Fcn1/1 -> Product2/2
  Theta/1 -> Relational Operator/1, Relational Operator1/1, Fcn/1, Relational Operator3/1, Fcn1/1, Relational Operator2/1, Scope/1
  Logical/1 -> Product2/1
  Fcn/1 -> Product1/2
  Logical Operator/1 -> Product1/1
  Relational Operator2/1 -> "not "/1, Logical/1
  not 1/1 -> Logical/2, Logical Operator/3
  "not "/1 -> Logical Operator/2
  Relational Operator3/1 -> not 1/1, Product3/2
  Relational Operator1/1 -> Logical Operator/1
  12.5 degree/1 -> Relational Operator3/2
  45 degree/1 -> Relational Operator2/2
  Constant1/1 -> Product/1, Product3/1
  Relational Operator/1 -> Product/2
  75 degree/1 -> Relational Operator1/2, Relational Operator/2
